simulink model "pardosealaschema"  (R2024b)
settings: Solver=VariableStepAuto  StartTime=0.0  StopTime=12000.0  RelTol=1e-3
values from neighbouring files (symbols this model uses):
  A = [-1/Tp 1/Tp ; kp/(kc*Tc) -((1+kp/kc)/Tc)]    [pardoseala.m]    (also in simulare.m = [-1/Ta -ke/La ; km/J 0]; tema1.m = [ k1*Ti*(kE2)/(2*Ti+1) 0 ; 0 k1*Ti*(kE1)/(2*Ti+1)])
  B = [ kE/(kp * Tp) 0 ; 0 1/Tc]    [pardoseala.m]    (also in simulare.m = [kE/La 0 ; 0 -1/J]; tema1.m = [ kC/Tc 0 ; 0 -Ti])
  C = [1 0 ; 0 1]    [pardoseala.m]    (also in simulare.m; tema1.m)
  D = [0 0 ; 0 0]    [pardoseala.m]    (also in simulare.m = zeros(2); tema1.m)
  kc = 125    [pardoseala.m]
  kE = 1000    [pardoseala.m]    (also in simulare.m = 42.85)
  kp = 500    [pardoseala.m]
  Tc = 300    [pardoseala.m]    (also in tema1.m = 0.5)
  Tp = 60    [pardoseala.m]
settings Model: Creator=albertrosca  LastModifiedBy=albertrosca

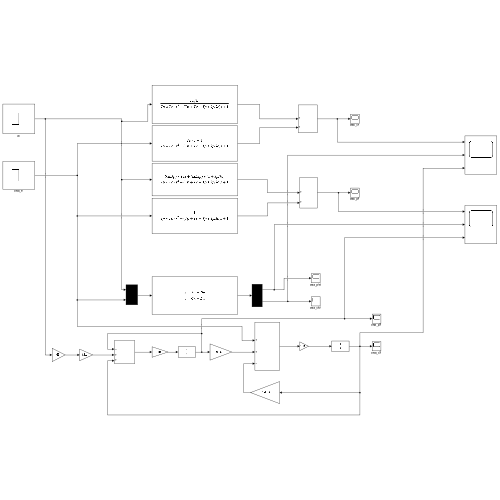
[thumbnail: Simulink's stored preview of the top-level diagram]
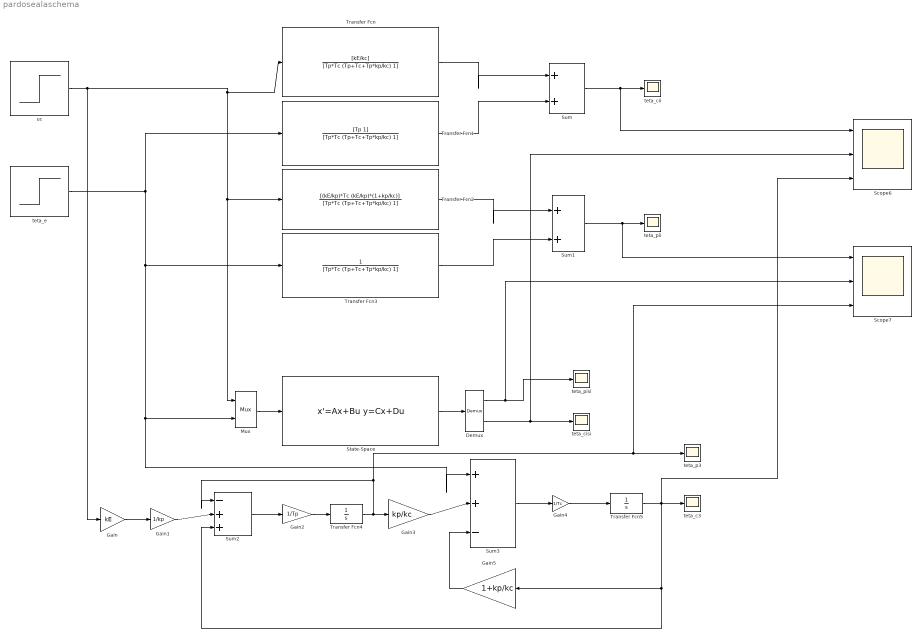
== system pardosealaschema ==
  Demux : Demux  Outputs=2
  Gain : Gain  Gain=kE
  Gain1 : Gain  Gain=1/kp
  Gain2 : Gain  Gain=1/Tp
  Gain3 : Gain  Gain=kp/kc
  Gain4 : Gain  Gain=1/Tc
  Gain5 : Gain  Gain=1+kp/kc
  Mux : Mux  Inputs=2
  Scope6 : Scope  NumInputPorts=3
  Scope7 : Scope  NumInputPorts=3
  State-Space : StateSpace  A=A  B=B  C=C  D=D  InitialCondition=0
  Sum : Sum  Inputs=|++
  Sum1 : Sum  Inputs=|++
  Sum2 : Sum  Inputs=|-++
  Sum3 : Sum  Inputs=|++-
  Transfer Fcn : TransferFcn  Numerator=[kE/kc]  Denominator=[Tp*Tc (Tp+Tc+Tp*kp/kc) 1]
  Transfer Fcn1 : TransferFcn  Numerator=[Tp 1]  Denominator=[Tp*Tc (Tp+Tc+Tp*kp/kc) 1]
  Transfer Fcn2 : TransferFcn  Numerator=[(kE/kp)*Tc (kE/kp)*(1+kp/kc)]  Denominator=[Tp*Tc (Tp+Tc+Tp*kp/kc) 1]
  Transfer Fcn3 : TransferFcn  Denominator=[Tp*Tc (Tp+Tc+Tp*kp/kc) 1]
  Transfer Fcn4 : TransferFcn  Denominator=[1 0]
  Transfer Fcn5 : TransferFcn  Denominator=[1 0]
  teta_c3 : Scope
  teta_cii : Scope
  teta_cisi : Scope
  teta_e : Step  Time=5000  After=-10  SampleTime=0
  teta_p3 : Scope
  teta_pii : Scope
  teta_pisi : Scope
  uc : Step  Time=0  After=2.5  SampleTime=0
  wires:
  uc/1 -> Transfer Fcn/1, Mux/1, Transfer Fcn2/1, Gain/1
  teta_e/1 -> Transfer Fcn1/1, Transfer Fcn3/1, Sum3/1, Mux/2
  Transfer Fcn/1 -> Sum/1
  Transfer Fcn1/1 -> Sum/2
  Transfer Fcn2/1 -> Sum1/1
  Transfer Fcn3/1 -> Sum1/2
  Sum1/1 -> Scope7/1, teta_pii/1
  Sum/1 -> Scope6/1, teta_cii/1
  Mux/1 -> State-Space/1
  State-Space/1 -> Demux/1
  Demux/1 -> Scope7/2, teta_pisi/1
  Demux/2 -> Scope6/2, teta_cisi/1
  Gain3/1 -> Sum3/2
  Sum2/1 -> Gain2/1
  Gain/1 -> Gain1/1
  Gain1/1 -> Sum2/2
  Gain2/1 -> Transfer Fcn4/1
  Transfer Fcn4/1 -> Scope7/3, teta_p3/1, Sum2/1, Gain3/1
  Sum3/1 -> Gain4/1
  Gain4/1 -> Transfer Fcn5/1
  Transfer Fcn5/1 -> Gain5/1, Sum2/3, Scope6/3, teta_c3/1
  Gain5/1 -> Sum3/3
